simulink model "TestLpe"  (R2020b)
settings: Solver=VariableStepAuto  StartTime=0.0  StopTime=60  RelTol=1e-3  EnableMultiTasking=on
InitFcn:
  | % load tfwt_00_run_01.mat
  | 
  | clear
  | load 2017-07-18-13-36-00_fullrate_left_right_yaw
  | if ~exist( 'logOriginal' )
  |     logOriginal = dataInOriginal
  | end
  | flog = logOriginal;
  | tSart = flog.vehicle_attitude.time(1);
  | timeStep = 0; %flog.vehicle_attitude.time(2) - flog.vehicle_attitude.time(1);
  | flog.sensor_combined.time = flog.sensor_combined.time - flog.vehicle_attitude.time(1) - timeStep;
  | flog.att_pos_mocap.time = flog.att_pos_mocap.time - flog.vehicle_attitude.time(1) - timeStep;
  | flog.control_state.time = flog.control_state.time - flog.vehicle_attitude.time(1) - timeStep;
  | flog.vehicle_local_position.time = flog.vehicle_local_position.time - flog.vehicle_attitude.time(1) - timeStep;
  | flog.vehicle_attitude.time = flog.vehicle_attitude.time - flog.vehicle_attitude.time(1);
  | 
  | tSimEnd = flog.vehicle_attitude.time(end);
(part 1 of 4)
settings Model: Creator=jban039  LastModifiedBy=jeremie
settings DataIOCC: LimitDataPoints=on
settings OptimizationCC: LifeSpan=inf
settings DebuggingCC: AllowSymbolicDim=off  SFUnexpectedBacktrackingDiag=warning  SFNoUnconditionalDefaultTransitionDiag=warning  SFExecutionAtInitializationDiag=none  ArithmeticOperatorsInVariantConditions=warning
settings ModelReferenceCC: PropagateSignalLabelsOutOfModel=off
settings SFSimCC: SimUseLocalCustomCode=off  CustomCodeUndefinedFunction=UseInterfaceOnly
settings RTWCC: RTWUseLocalCustomCode=off
settings CodeAppCC: StateflowObjectComments=on
settings GRTTargetCC: TargetLangStandard=C89/C90 (ANSI)
settings ConfigComp: CovMetricSettings=dw  CovSaveCumulativeToWorkspaceVar=on  CovSaveSingleToWorkspaceVar=on  CovExternalEMLEnable=off

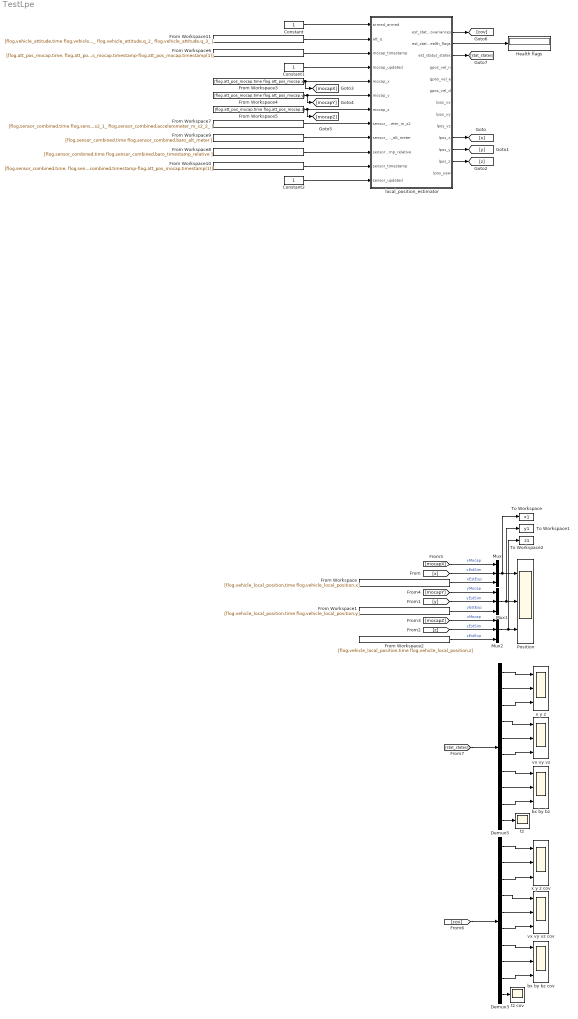
== system TestLpe ==
  Constant : Constant
  Constant1 : Constant
  Constant2 : Constant
  Demux3 : Demux  Outputs=10
  Demux5 : Demux  Outputs=10
  From Workspace : FromWorkspace  VariableName=[flog.vehicle_local_position.time flog.vehicle_local_position.x]  Interpolate=off  OutputAfterFinalValue=Holding final value
  From Workspace1 : FromWorkspace  VariableName=[flog.vehicle_local_position.time flog.vehicle_local_position.y]  Interpolate=off  OutputAfterFinalValue=Holding final value
  From Workspace10 : FromWorkspace  VariableName=[flog.sensor_combined.time, flog.sensor_combined.timestamp-flog.att_pos_mocap.timestamp(1)]  Interpolate=off  OutputAfterFinalValue=Holding final value
  From Workspace11 : FromWorkspace  VariableName=[flog.vehicle_attitude.time flog.vehicle_attitude.q_0_ flog.vehicle_attitude.q_1_ flog.vehicle_attitude.q_2_ flog.vehicle_attitude.q_3_ ]  Interpolate=off  OutputAfterFinalValue=Holding final value
  From Workspace2 : FromWorkspace  VariableName=[flog.vehicle_local_position.time flog.vehicle_local_position.z]  Interpolate=off  OutputAfterFinalValue=Holding final value
  From Workspace3 : FromWorkspace  VariableName=[flog.att_pos_mocap.time flog.att_pos_mocap.x]  Interpolate=off  OutputAfterFinalValue=Holding final value
  From Workspace4 : FromWorkspace  VariableName=[flog.att_pos_mocap.time flog.att_pos_mocap.y]  Interpolate=off  OutputAfterFinalValue=Holding final value
  From Workspace5 : FromWorkspace  VariableName=[flog.att_pos_mocap.time flog.att_pos_mocap.z]  Interpolate=off  OutputAfterFinalValue=Holding final value
  From Workspace6 : FromWorkspace  VariableName=[flog.att_pos_mocap.time, flog.att_pos_mocap.timestamp-flog.att_pos_mocap.timestamp(1)]  Interpolate=off  OutputAfterFinalValue=Holding final value
  From Workspace7 : FromWorkspace  VariableName=[flog.sensor_combined.time flog.sensor_combined.accelerometer_m_s2_0_ flog.sensor_combined.accelerometer_m_s2_1_ flog.sensor_combined.accelerometer_m_s2_2_ ]  Interpolate=off  OutputAfterFinalValue=Holding final value
  From Workspace8 : FromWorkspace  VariableName=[flog.sensor_combined.time flog.sensor_combined.baro_timestamp_relative ]  Interpolate=off  OutputAfterFinalValue=Holding final value
  From Workspace9 : FromWorkspace  VariableName=[flog.sensor_combined.time flog.sensor_combined.baro_alt_meter ]  Interpolate=off  OutputAfterFinalValue=Holding final value
  Health flags : Display
  Mux : Mux  Inputs=3
  Mux1 : Mux  Inputs=3
  Mux2 : Mux  Inputs=3
  Position : Scope  NumInputPorts=3
  To Workspace : ToWorkspace  VariableName=x1  SaveFormat=Structure With Time  SampleTime=-1
  To Workspace1 : ToWorkspace  VariableName=y1  SaveFormat=Structure With Time  SampleTime=-1
  To Workspace2 : ToWorkspace  VariableName=z1  SaveFormat=Structure With Time  SampleTime=-1
  bx by bz : Scope  NumInputPorts=3
  bx by bz cov : Scope  NumInputPorts=3
  local_position_estimator : Subsystem  AncestorBlock=Px4Library/local_position_estimator  mask(PX4 LPE (local position estimator): local_position_estimator){LPE_SAMPLING_PERIOD=0.01, LPE_ACC_XY=0.012, LPE_ACC_Z=0.02, LPE_BAR_Z=3, LPE_EPH_MAX=3, LPE_EPV_MAX=5, LPE_FAKE_ORIGIN=0, LPE_FGYRO_HP=0.001, LPE_FLW_OFF_Z=0, LPE_FLW_QMIN=150, LPE_FLW_R=7, LPE_FLW_RR=7, LPE_FLW_SCALE=1.3, LPE_GPS_DELAY=0.29, LPE_GPS_VXY=0.25, LPE_GPS_VZ=0.25, LPE_GPS_XY=1, LPE_GPS_Z=3, LPE_LAND_VXY=0.05, LPE_LAND_Z=0.03, LPE_LAT=47.3977, LPE_LDR_OFF_Z=0, LPE_LDR_Z=0.03, LPE_LON=8.5456, LPE_PN_B=0.001, LPE_PN_P=0.1, LPE_PN_T=0.001, LPE_PN_V=0.1, LPE_SNR_OFF_Z=0, LPE_SNR_Z=0.05, LPE_T_MAX_GRADE=1, LPE_VIC_P=0.001, LPE_VIS_DELAY=0.1, LPE_VIS_XY=0.1, LPE_VIS_Z=0.5, LPE_VXY_PUB=0.3, LPE_X_LP=5, LPE_Z_PUB=1, LPE_FUSION=64, Barometer=off, GPS=off, LIDAR=off, Flow=off, Sonar=off, Vision=off, Mocap=on, Land=off}
      mask prompts: LPE_SAMPLING_PERIOD "Sampling period (s)"; LPE_ACC_XY "LPE_ACC_XY - Accelerometer xy noise density (m/s^2/sqrt(Hz))"; LPE_ACC_Z "LPE_ACC_Z - Accelerometer z noise density (m/s^2/sqrt(Hz))"; LPE_BAR_Z "LPE_BAR_Z - Barometric presssure altitude z standard deviation. (m)"; LPE_EPH_MAX "LPE_EPH_MAX - Max EPH allowed for GPS initialization (m)"; LPE_EPV_MAX "LPE_EPV_MAX - Max EPV allowed for GPS initialization (m)"; LPE_FAKE_ORIGIN "LPE_FAKE_ORIGIN - Enable publishing of a fake global position (e.g for AUTO missions using Optical Flow) (-)"; LPE_FGYRO_HP "LPE_FGYRO_HP - Flow gyro high pass filter cut off frequency (Hz)"; LPE_FLW_OFF_Z "LPE_FLW_OFF_Z - Optical flow z offset from center (m)"; LPE_FLW_QMIN "LPE_FLW_QMIN - Optical flow minimum quality threshold (-)"; LPE_FLW_R "LPE_FLW_R - Optical flow rotation (roll/pitch) noise gain (m/s / (rad))"; LPE_FLW_RR "LPE_FLW_RR - Optical flow angular velocity noise gain (m/s / (rad/s))"; LPE_FLW_SCALE "LPE_FLW_SCALE - Optical flow scale (m)"; LPE_GPS_DELAY "LPE_GPS_DELAY - GPS delay compensaton (sec)"; LPE_GPS_VXY "LPE_GPS_VXY - GPS xy velocity standard deviation. (m/s)"; LPE_GPS_VZ "LPE_GPS_VZ - GPS z velocity standard deviation. (m/s)"; LPE_GPS_XY "LPE_GPS_XY - Minimum GPS xy standard deviation, uses reported EPH if greater. (m)"; LPE_GPS_Z "LPE_GPS_Z - Minimum GPS z standard deviation, uses reported EPV if greater. (m)"; LPE_LAND_VXY "LPE_LAND_VXY - Land detector xy velocity standard deviation (m/s)"; LPE_LAND_Z "LPE_LAND_Z - Land detector z standard deviation (m)"; LPE_LAT "LPE_LAT - Local origin latitude for nav w/o GPS (deg)"; LPE_LDR_OFF_Z "LPE_LDR_OFF_Z - Lidar z offset from center of vehicle +down (m)"; LPE_LDR_Z "LPE_LDR_Z - Lidar z standard deviation. (m)"; LPE_LON "LPE_LON - Local origin longitude for nav w/o GPS (deg)"; LPE_PN_B "LPE_PN_B - Accel bias propagation noise density ((m/s^2)/s/sqrt(Hz))"; LPE_PN_P "LPE_PN_P - Position propagation noise density (m/s/sqrt(Hz))"; LPE_PN_T "LPE_PN_T - Terrain random walk noise density, hilly/outdoor (0.1), flat/Indoor (0.001) ((m/s)/(sqrt(hz)))"; LPE_PN_V "LPE_PN_V - Velocity propagation noise density ((m/s)/s/sqrt(Hz))"; LPE_SNR_OFF_Z "LPE_SNR_OFF_Z - Sonar z offset from center of vehicle +down (m)"; LPE_SNR_Z "LPE_SNR_Z - Sonar z standard deviation. (m)"; LPE_T_MAX_GRADE "LPE_T_MAX_GRADE - Terrain maximum percent grade, hilly/outdoor (100 = 45 deg), flat/Indoor (0 = 0 deg) (%)"; LPE_VIC_P "LPE_VIC_P - Vicon position standard deviation. (m)"; LPE_VIS_DELAY "LPE_VIS_DELAY - Vision delay compensaton. (sec)"; LPE_VIS_XY "LPE_VIS_XY - Vision xy standard deviation. (m)"; LPE_VIS_Z "LPE_VIS_Z - Vision z standard deviation. (m)"; LPE_VXY_PUB "LPE_VXY_PUB - Required velocity xy standard deviation to publish position (m/s)"; LPE_X_LP "LPE_X_LP - Cut frequency for state publication (Hz)"; LPE_Z_PUB "LPE_Z_PUB - Required z standard deviation to publish altitude/ terrain (m)"; LPE_FUSION "LPE_FUSION - Integer bitmask controlling data fusion (-)"; Barometer "Use Barometer"; GPS "Use GPS"; LIDAR "Use LIDAR"; Flow "Use Flow"; Sonar "Use Sonar"; Vision "Use Vision"; Mocap "Use Mocap"; Land "Use Land"
      mask Callback Barometer:
      | status = get_param( gcb, 'Barometer' );
      | if strcmp( status, 'on' )
      | 	lpe = bitor( uint8(str2num(get_param( gcb, 'LPE_FUSION' ))), uint8(2^0) );
      | 	set_param( gcb, 'LPE_FUSION', num2str(lpe) );
      | else
      | 	lpe = bitand( uint8(str2num(get_param( gcb, 'LPE_FUSION' ))), bitcmp(uint8(2^0), 'uint8' ));
      | 	set_param( gcb, 'LPE_FUSION', num2str(lpe) );
      | end
      mask Callback GPS:
      | status = get_param( gcb, 'GPS' );
      | if strcmp( status, 'on' )
      | 	lpe = bitor( uint8(str2num(get_param( gcb, 'LPE_FUSION' ))), uint8(2^1) );
      | 	set_param( gcb, 'LPE_FUSION', num2str(lpe) );
      | else
      | 	lpe = bitand( uint8(str2num(get_param( gcb, 'LPE_FUSION' ))), bitcmp(uint8(2^1), 'uint8' ));
      | 	set_param( gcb, 'LPE_FUSION', num2str(lpe) );
      | end
      mask Callback LIDAR:
      | status = get_param( gcb, 'LIDAR' );
      | if strcmp( status, 'on' )
      | 	lpe = bitor( uint8(str2num(get_param( gcb, 'LPE_FUSION' ))), uint8(2^2) );
      | 	set_param( gcb, 'LPE_FUSION', num2str(lpe) );
      | else
      | 	lpe = bitand( uint8(str2num(get_param( gcb, 'LPE_FUSION' ))), bitcmp(uint8(2^2), 'uint8' ));
      | 	set_param( gcb, 'LPE_FUSION', num2str(lpe) );
      | end
      mask Callback Flow:
      | status = get_param( gcb, 'Flow' );
      | if strcmp( status, 'on' )
      | 	lpe = bitor( uint8(str2num(get_param( gcb, 'LPE_FUSION' ))), uint8(2^3) );
      | 	set_param( gcb, 'LPE_FUSION', num2str(lpe) );
      | else
      | 	lpe = bitand( uint8(str2num(get_param( gcb, 'LPE_FUSION' ))), bitcmp(uint8(2^3), 'uint8' ));
      | 	set_param( gcb, 'LPE_FUSION', num2str(lpe) );
      | end
      mask Callback Sonar:
      | status = get_param( gcb, 'Sonar' );
      | if strcmp( status, 'on' )
      | 	lpe = bitor( uint8(str2num(get_param( gcb, 'LPE_FUSION' ))), uint8(2^4) );
      | 	set_param( gcb, 'LPE_FUSION', num2str(lpe) );
      | else
      | 	lpe = bitand( uint8(str2num(get_param( gcb, 'LPE_FUSION' ))), bitcmp(uint8(2^4), 'uint8' ));
      | 	set_param( gcb, 'LPE_FUSION', num2str(lpe) );
      | end
      mask Callback Vision:
      | status = get_param( gcb, 'Vision' );
      | if strcmp( status, 'on' )
      | 	lpe = bitor( uint8(str2num(get_param( gcb, 'LPE_FUSION' ))), uint8(2^5) );
      | 	set_param( gcb, 'LPE_FUSION', num2str(lpe) );
      | else
      | 	lpe = bitand( uint8(str2num(get_param( gcb, 'LPE_FUSION' ))), bitcmp(uint8(2^5), 'uint8' ));
      | 	set_param( gcb, 'LPE_FUSION', num2str(lpe) );
      | end
      mask Callback Mocap:
      | status = get_param( gcb, 'Mocap' );
      | if strcmp( status, 'on' )
      | 	lpe = bitor( uint8(str2num(get_param( gcb, 'LPE_FUSION' ))), uint8(2^6) );
      | 	set_param( gcb, 'LPE_FUSION', num2str(lpe) );
      | else
      | 	lpe = bitand( uint8(str2num(get_param( gcb, 'LPE_FUSION' ))), bitcmp(uint8(2^6), 'uint8' ));
      | 	set_param( gcb, 'LPE_FUSION', num2str(lpe) );
      | end
      mask Callback Land:
      | status = get_param( gcb, 'Land' );
      | if strcmp( status, 'on' )
      | 	lpe = bitor( uint8(str2num(get_param( gcb, 'LPE_FUSION' ))), uint8(2^7) );
      | 	set_param( gcb, 'LPE_FUSION', num2str(lpe) );
      | else
      | 	lpe = bitand( uint8(str2num(get_param( gcb, 'LPE_FUSION' ))), bitcmp(uint8(2^7), 'uint8' ));
      | 	set_param( gcb, 'LPE_FUSION', num2str(lpe) );
      | end
  tz : Scope
  tz cov : Scope
  vx vy vz : Scope  NumInputPorts=3
  vx vy vz cov : Scope  NumInputPorts=3
  x y z : Scope  NumInputPorts=3
  x y z cov : Scope  NumInputPorts=3
  wires:
  Mux1/1 -> To Workspace1/1, Position/2
  Mux/1 -> To Workspace/1, Position/1
  Mux2/1 -> To Workspace2/1, Position/3
  Demux5/2 -> x y z/2
  Demux5/1 -> x y z/1
  Demux5/3 -> x y z/3
  Demux5/4 -> vx vy vz/1
  Demux5/5 -> vx vy vz/2
  Demux5/6 -> vx vy vz/3
  Demux5/7 -> bx by bz/1
  Demux5/8 -> bx by bz/2
  Demux5/9 -> bx by bz/3
  Demux5/10 -> tz/1
  [stat_states] -> Demux5/1
  Demux3/2 -> x y z cov/2
  Demux3/1 -> x y z cov/1
  Demux3/3 -> x y z cov/3
  Demux3/4 -> vx vy vz cov/1
  Demux3/5 -> vx vy vz cov/2
  Demux3/6 -> vx vy vz cov/3
  Demux3/7 -> bx by bz cov/1
  Demux3/8 -> bx by bz cov/2
  Demux3/9 -> bx by bz cov/3
  Demux3/10 -> tz cov/1
  [cov] -> Demux3/1
  local_position_estimator/2(est_status_health_flags) -> Health flags/1
  local_position_estimator/10(lpos_x) -> [x]
  local_position_estimator/11(lpos_y) -> [y]
  local_position_estimator/12(lpos_z) -> [z]
  From Workspace1/1 -> Mux1/3  "yEstExp"
  From Workspace2/1 -> Mux2/3  "zEstExp"
  From Workspace/1 -> Mux/3  "xEstExp"
  [x] -> Mux/2  "xEstSim"
  [y] -> Mux1/2  "yEstSim"
  [z] -> Mux2/2  "zEstSim"
  From Workspace3/1 -> local_position_estimator/5(mocap_x), [mocapX]
  From Workspace5/1 -> local_position_estimator/7(mocap_z), [mocapZ]
  From Workspace4/1 -> local_position_estimator/6(mocap_y), [mocapY]
  From Workspace6/1 -> local_position_estimator/3(mocap_timestamp)
  Constant/1 -> local_position_estimator/1(armed_armed)
  [mocapX] -> Mux/1  "xMocap"
  [mocapY] -> Mux1/1  "yMocap"
  [mocapZ] -> Mux2/1  "zMocap"
  Constant1/1 -> local_position_estimator/4(mocap_updated)
  From Workspace7/1 -> local_position_estimator/8(sensor_accelerometer_m_s2)
  From Workspace8/1 -> local_position_estimator/10(sensor_baro_timestamp_relative)
  From Workspace9/1 -> local_position_estimator/9(sensor_baro_alt_meter)
  From Workspace10/1 -> local_position_estimator/11(sensor_timestamp)
  Constant2/1 -> local_position_estimator/12(sensor_updated)
  From Workspace11/1 -> local_position_estimator/2(att_q)
  local_position_estimator/3(est_status_states) -> [stat_states]
  local_position_estimator/1(est_status_covariances) -> [cov]

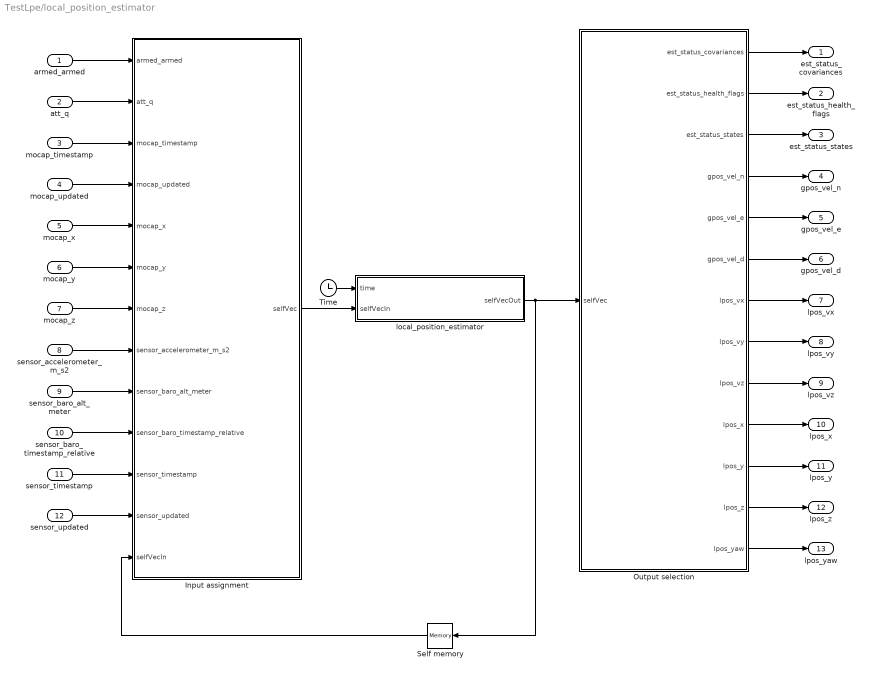
== system TestLpe/local_position_estimator ==
  armed_armed : Inport
  att_q : Inport  Port=2
  mocap_timestamp : Inport  Port=3
  mocap_updated : Inport  Port=4
  mocap_x : Inport  Port=5
  mocap_y : Inport  Port=6
  mocap_z : Inport  Port=7
  sensor_accelerometer_m_s2 : Inport  Port=8
  sensor_baro_alt_meter : Inport  Port=9
  sensor_baro_timestamp_relative : Inport  Port=10
  sensor_timestamp : Inport  Port=11
  sensor_updated : Inport  Port=12
  Input assignment : MATLAB Function  TreatAsAtomicUnit=on
  Output selection : MATLAB Function  TreatAsAtomicUnit=on
  Self memory : Memory  InitialCondition=[0, 0, 0, 0, 0, 0, 0, 0, 0, 0, 0, 0, 0, 0, 0, 0, 0, 0, 0, 0, 0, 0, 0, 0, 0, 0, 0, 0, 0, 0, 0, 0, 0, 0, 0, 0, 0, 0, 0, 0, 0, 0, 0, 0, 0, 0, 0, 0, 0, 0, 0, 0, 0, 0, 0, 0, 0, 0, 0, 0, 0, 0, 0, 0, 0, 0, 0, 0, 0, 0, 0, 0, 0, 0, 0, 0, 0, 0, 0, 0, 0, 0, 0, 0, 0, 0, 0, 0, 0, 0, 0, 0, 0, 0, 0, 0, 0, 0, 0, 0, 0, 0, 0, 0, 0, 0, 0, 0, 0, 0, 0, 0, 0, 0, 0, 0, 0, 0, 0, 0, 0, 0, 0, 0, 0, 0, 0, 0, 0, 0, 0, 8.82050518214, 12.094592431, 13.9876612368, 16.0875642296, 17.8797700658, 19.6465647819, 1e-1, 2.0, 2.0, 2.0, 2^2, 2^0, 2^1, 2^7, 2^1, 2^6, 2^0, 2^4, 2^5, 2^2, 2^3, 0, 10.0, 8, 0, 0, 0, 0, 0, 0, 0, 0, 0, 0, 8, 0, 0, 0, 0, 0, 0, 0, 0, 0, 0, 8, 0, 0, 0, 0, 0, 0, 0, 0, 0, 0, 2*LPE_VXY_PUB*LPE_VXY_PUB, 0, 0, 0, 0, 0, 0, 0, 0, 0, 0, 2*LPE_VXY_PUB*LPE_VXY_PUB, 0, 0, 0, 0, 0, 0, 0, 0, 0, 0, 2*LPE_VXY_PUB*LPE_VXY_PUB, 0, 0, 0, 0, 0, 0, 0, 0, 0, 0, 1e-6, 0, 0, 0, 0, 0, 0, 0, 0, 0, 0, 1e-6, 0, 0, 0, 0, 0, 0, 0, 0, 0, 0, 1e-6, 0, 0, 0, 0, 0, 0, 0, 0, 0, 0, 8, 1.0e6, 0, 0, 0, 0, 0, 0, 0, 0, 0, 0, 0, 0, 0, 0, 0, 0, 0, 0, 0, 0, 0, 0, 0, 0, 0, 0, 0, 0, 0, 0, 0, 0, 0, 0, 0, 0, 0, 0, 0, 0, 0, 0, 0, 0, 0, 0, 0, 0, 0, 0, 0, 0, 0, 0, 0, 0, 0, 0, 0, 0, 0, 0, 0, 0, 0, 0, 0, 0, 0, 0, 0, 0, 0, 0, 0, 0, 0, 0, 0, 0, 0, 0, 0, 0, 0, 0, 0, 0, 0, 0, 0, 0, 0, 0, 0, 0, 0, 0, 0, 0, 0, 0, 0, 0, 0, 0, 0, 0, 0, 0, 0, 0, 0, 0, 0, 0, 0, 0, 2^0, 2^3, 2^1, 2^7, 2^2, 2^6, 2^4, 2^5, 0, LPE_ACC_XY, 0, LPE_ACC_Z, LPE_SAMPLING_PERIOD, LPE_X_LP, 0, 0, 0, 0, 0, 0, LPE_BAR_Z, LPE_SAMPLING_PERIOD, 0, 0, 0, 0, LPE_FAKE_ORIGIN, 0, LPE_FGYRO_HP, LPE_FGYRO_HP, LPE_FLW_QMIN, LPE_FLW_R, LPE_FLW_RR, LPE_FLW_SCALE, LPE_FLW_OFF_Z, LPE_FUSION, 0, LPE_GPS_DELAY, LPE_EPH_MAX, LPE_EPV_MAX, LPE_GPS_VXY, LPE_GPS_VZ, LPE_GPS_XY, LPE_GPS_Z, LPE_LAT, LPE_LON, 0, 0, LPE_LAND_VXY, LPE_LAND_Z, 0, LPE_LDR_OFF_Z, LPE_LDR_Z, 0, 0, 0, 0, 0, 0, 0, LPE_VIC_P, LPE_PN_B, LPE_PN_P, LPE_PN_T, LPE_PN_V, 8, 0, 0, 0, 0, 0, 0, 0, 0, 0, 0, 0, 0, 0, 0, 0, 0, 0, 0, 0, 0, 0, 0, 0, 0, 0, 0, 0, 0, 0, 0, 0, 0, 0, 0, 0, 0, 0, 0, 0, 0, 0, 0, 0, 0, 0, 0, 0, 0, 0, 0, 0, 0, 0, 0, 0, 0, 0, 0, 0, 0, 0, 0, 0, 0, 0, 0, 0, 0, 0, 0, 0, 0, 0, 0, 255, 0, LPE_SNR_OFF_Z, LPE_SNR_Z, 0, 0, 0, 0, 0, 0, 0, 0, 0, 0, 0, 0, 0, 0, 0, 0, 0, 0, 0, 0, 0, 0, 0, 0, 0, 0, 0, 0, 0, 0, 0, 0, 0, 0, 0, 0, 0, 0, 0, 1, 1, LPE_T_MAX_GRADE, 0, 0, 0, 0, 0, 0, 0, 0, 0, 0, 0, LPE_VIS_DELAY, LPE_VIS_XY, LPE_VIS_Z, LPE_VXY_PUB, 0, 0, 0, 0, 0, 0, 0, 0, 0, 0, 0, 0, 0, 0, 0, 0, 0, 0, 0, 0, 0, 0, 0, 0, 0, 0, 0, 0, 0, 0, 0, 0, 0, 0, 0, 0, 0, 0, 0, 0, 0, 0, 0, 0, 0, 0, 0, 0, 0, 0, 0, 0, 0, 0, 0, 0, 0, 0, 0, 0, 0, 0, 0, 0, 0, 0, 0, 0, 0, 0, 0, 0, 0, 0, 0, 0, 0, 0, 0, 0, 0, 0, 0, 0, 0, 0, 0, 0, 0, 0, 0, 0, 0, 0, 0, 0, 0, 0, 0, 0, 0, 0, 0, 0, 0, 0, 0, 0, 0, 0, 1, 1, LPE_SAMPLING_PERIOD, LPE_X_LP, 0, 0, 0, 0, 0, 0, 0, 0, 0, 0, LPE_Z_PUB]
  Time : Clock
  local_position_estimator : MATLAB Function  TreatAsAtomicUnit=on  SystemSampleTime=LPE_SAMPLING_PERIOD
  est_status_covariances : Outport  VectorParamsAs1DForOutWhenUnconnected=off
  est_status_health_flags : Outport  Port=2  VectorParamsAs1DForOutWhenUnconnected=off
  est_status_states : Outport  Port=3  VectorParamsAs1DForOutWhenUnconnected=off
  gpos_vel_n : Outport  Port=4  VectorParamsAs1DForOutWhenUnconnected=off
  gpos_vel_e : Outport  Port=5  VectorParamsAs1DForOutWhenUnconnected=off
  gpos_vel_d : Outport  Port=6  VectorParamsAs1DForOutWhenUnconnected=off
  lpos_vx : Outport  Port=7  VectorParamsAs1DForOutWhenUnconnected=off
  lpos_vy : Outport  Port=8  VectorParamsAs1DForOutWhenUnconnected=off
  lpos_vz : Outport  Port=9  VectorParamsAs1DForOutWhenUnconnected=off
  lpos_x : Outport  Port=10  VectorParamsAs1DForOutWhenUnconnected=off
  lpos_y : Outport  Port=11  VectorParamsAs1DForOutWhenUnconnected=off
  lpos_z : Outport  Port=12  VectorParamsAs1DForOutWhenUnconnected=off
  lpos_yaw : Outport  Port=13  VectorParamsAs1DForOutWhenUnconnected=off
  wires:
  Output selection/13(lpos_yaw) -> lpos_yaw/1
  Output selection/12(lpos_z) -> lpos_z/1
  Output selection/11(lpos_y) -> lpos_y/1
  Output selection/10(lpos_x) -> lpos_x/1
  Output selection/9(lpos_vz) -> lpos_vz/1
  Output selection/8(lpos_vy) -> lpos_vy/1
  Output selection/7(lpos_vx) -> lpos_vx/1
  Output selection/6(gpos_vel_d) -> gpos_vel_d/1
  Output selection/5(gpos_vel_e) -> gpos_vel_e/1
  Output selection/4(gpos_vel_n) -> gpos_vel_n/1
  Output selection/3(est_status_states) -> est_status_states/1
  Output selection/2(est_status_health_flags) -> est_status_health_flags/1
  Output selection/1(est_status_covariances) -> est_status_covariances/1
  sensor_updated/1 -> Input assignment/12(sensor_updated)
  sensor_timestamp/1 -> Input assignment/11(sensor_timestamp)
  sensor_baro_timestamp_relative/1 -> Input assignment/10(sensor_baro_timestamp_relative)
  sensor_baro_alt_meter/1 -> Input assignment/9(sensor_baro_alt_meter)
  sensor_accelerometer_m_s2/1 -> Input assignment/8(sensor_accelerometer_m_s2)
  mocap_z/1 -> Input assignment/7(mocap_z)
  mocap_y/1 -> Input assignment/6(mocap_y)
  mocap_x/1 -> Input assignment/5(mocap_x)
  mocap_updated/1 -> Input assignment/4(mocap_updated)
  mocap_timestamp/1 -> Input assignment/3(mocap_timestamp)
  att_q/1 -> Input assignment/2(att_q)
  armed_armed/1 -> Input assignment/1(armed_armed)
  Time/1 -> local_position_estimator/1(time)
  Self memory/1 -> Input assignment/13(selfVecIn)
  local_position_estimator/1(selfVecOut) -> Self memory/1, Output selection/1(selfVec)
  Input assignment/1(selfVec) -> local_position_estimator/2(selfVecIn)

== matlab function TestLpe/local_position_estimator/Input assignment ==
  data: armed_armed input; att_q input; mocap_timestamp input; mocap_updated input; mocap_x input; mocap_y input; mocap_z input; sensor_accelerometer_m_s2 input; sensor_baro_alt_meter input; sensor_baro_timestamp_relative input; sensor_timestamp input; sensor_updated input; selfVecIn input; selfVec output
function selfVec = InputAssignment( ...
	                             armed_armed, ...
	                                   att_q, ...
	                         mocap_timestamp, ...
	                           mocap_updated, ...
	                                 mocap_x, ...
	                                 mocap_y, ...
	                                 mocap_z, ...
	               sensor_accelerometer_m_s2, ...
	                   sensor_baro_alt_meter, ...
	          sensor_baro_timestamp_relative, ...
	                        sensor_timestamp, ...
	                          sensor_updated, ...
	                               selfVecIn ...
	)
%#codegen

	selfVec = selfVecIn;

	% Variable assignment
	selfVec(518:518) =                              armed_armed;
	selfVec(519:522) =                                    att_q;
	selfVec(530:530) =                          mocap_timestamp;
	selfVec(531:531) =                            mocap_updated;
	selfVec(532:532) =                                  mocap_x;
	selfVec(533:533) =                                  mocap_y;
	selfVec(534:534) =                                  mocap_z;
	selfVec(537:539) =                sensor_accelerometer_m_s2;
	selfVec(540:540) =                    sensor_baro_alt_meter;
	selfVec(541:541) =           sensor_baro_timestamp_relative;
	selfVec(542:542) =                         sensor_timestamp;
	selfVec(543:543) =                           sensor_updated;
end
